simulink model "w1p4_mod"  (R2020a)
settings: Solver=VariableStepAuto  StartTime=0.0  StopTime=100  RelTol=1e-3
settings Model: Creator=avn19  LastModifiedBy=avn19

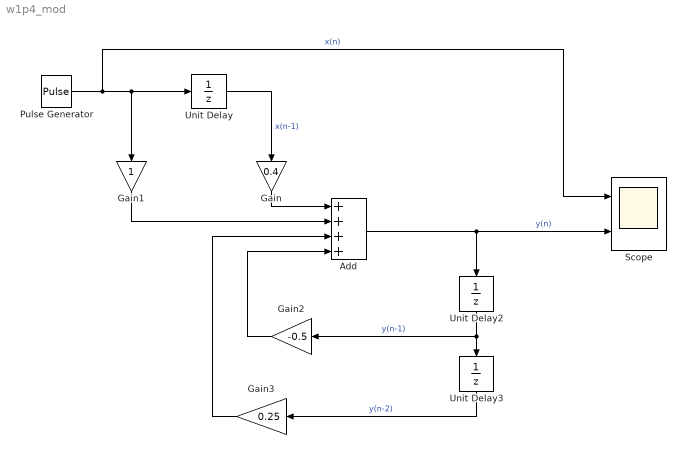
== system w1p4_mod ==
  Add : Sum  Inputs=++++
  Gain : Gain  Gain=0.4
  Gain1 : Gain
  Gain2 : Gain  Gain=-0.5
  Gain3 : Gain  Gain=0.25
  Pulse Generator : DiscretePulseGenerator  PulseType=Time based  Period=10  PulseWidth=5
  Scope : Scope  NumInputPorts=2
  Unit Delay : UnitDelay  SampleTime=-1  HasFrameUpgradeWarning=on
  Unit Delay2 : UnitDelay  SampleTime=-1  HasFrameUpgradeWarning=on
  Unit Delay3 : UnitDelay  SampleTime=-1  HasFrameUpgradeWarning=on
  wires:
  Pulse Generator/1 -> Unit Delay/1, Gain1/1, Scope/1  "x(n)"
  Unit Delay/1 -> Gain/1  "x(n-1)"
  Gain/1 -> Add/1
  Gain1/1 -> Add/2
  Add/1 -> Unit Delay2/1, Scope/2  "y(n)"
  Gain2/1 -> Add/4
  Gain3/1 -> Add/3
  Unit Delay2/1 -> Unit Delay3/1, Gain2/1  "y(n-1)"
  Unit Delay3/1 -> Gain3/1  "y(n-2)"
